simulink model "controller"  (Simulink 7.8)
settings: Solver=ode5  SolverMode=SingleTasking  StartTime=0.0  StopTime=50  FixedStep=0.01  RelTol=1e-3  AbsTol=1e-6
model workspace (MAT data in the model file):
  converter_data = [0  137.465208994  2.232; 0.1  137.065019157  2.075; 0.2  135.864449646  1.975; 0.3  135.664354728  1.846; 0.4  137.565256453  1.72; 0.5  140.366585312  1.564; 0.6  145.268910814  1.409; 0.7  152.872517717  1.254; 0.8  162.9773111  1.096; 0.81  164.27792807  1.08; 0.82  166.178829795  1.061; 0.83  167.979684062  1.043; 0.84  170.080680706  1.028; 0.85  172.781962105  1.012; 0.86  175.383196045  1.002; 0.87  179.585189333  1.002; 0.88  183.587087703  1.001; 0.89  189.890077635  0.998; 0.9  197.693779455  0.999; 0.92  215.902417037  1.001; 0.94  244.515990379  1.002]
  emap = [-40  -44  -49  -53  -57  -61  -65  -70  -74  -78  -82; 215  117  85  66  44  29  10  -2  -13  -22  -32; 245  208  178  148  122  104  85  66  48  33  18; 264  260  241  219  193  167  152  133  119  96  85; 264  279  282  275  260  238  223  208  189  171  152; 267  290  293  297  290  275  260  256  234  212  193; 267  297  305  305  305  301  293  282  267  249  226; 267  301  308  312  319  323  319  316  297  279  253; 267  301  312  319  327  327  327  327  312  293  267; 267  301  312  319  327  334  334  334  319  305  275]
  Iei = 0.0219914882836
  nevec = [800 1200 1600 2000 2400 2800 3200 3600 4000 4400 4800]
  p0 = 0.07934
  p1 = 0.07934
  thvec = [0; 20; 30; 40; 50; 60; 70; 80; 90; 100]
  vehicledata : num (value not decoded)
values from neighbouring files (symbols this model uses):
  downtab = [0 5 20 35 ... (first row only)    [transmission_data.m]
  downth = [0; 5; 40; 50; 90; 100]    [transmission_data.m]
  uptab = [10 30 50 1.0E+6 ... (first row only)    [transmission_data.m]
  upth = [0; 25; 35; 50; 90; 100]    [transmission_data.m]
Description:
  | ƒRƒ“ƒgƒ??[ƒ‰?eƒ‚ƒfƒ‹
settings Model: Creator=The MathWorks Inc.  LastModifiedBy=itoy  CovMetricSettings=dcmtr  CovHTMLOptions=-aTS=1 -bRG=1 -bTC=1 -hTR=0 -nFC=0 -scm=1 -bcm=1 -xEv=0  ExtModeTrigMode=oneshot  ExtModeArmWhenConnect=off  ExtModeAutoUpdateStatusClock=off
settings DataIOCC: LimitDataPoints=off  SaveOutput=off  SaveTime=off  SignalLoggingName=sigsOut
settings OptimizationCC: InlineParams=on  UseIntDivNetSlope=on  InlineInvariantSignals=on  InitFltsAndDblsToZero=on  EfficientMapNaN2IntZero=off  OptimizeModelRefInitCode=on  LifeSpan=1
settings DebuggingCC: SignalInfNanChecking=error  SaveWithParameterizedLinksMsg=none  CheckExecutionContextPreStartOutputMsg=on  CheckExecutionContextRuntimeOutputMsg=on  SolverPrmCheckMsg=none  MultiTaskDSMMsg=warning  MultiTaskCondExecSysMsg=none  IntegerOverflowMsg=error  FcnCallInpInsideContextMsg=Use local settings  BusObjectLabelMismatch=error  RootOutportRequireBusObject=error  StrictBusMsg=ErrorOnBusTreatedAsVector  BusNameAdapt=ErrorWithoutRepair  NonBusSignalsTreatedAsBus=error
settings HardwareCC: ProdIntDivRoundTo=Zero  ProdEndianess=LittleEndian  ProdHWDeviceType=NEC->V850  TargetIntDivRoundTo=Zero  TargetEndianess=LittleEndian  TargetHWDeviceType=MATLAB Host
settings ModelReferenceCC: ModelReferenceNumInstancesAllowed=Single
settings SFSimCC: SFSimEcho=off  SimParseCustomCode=off
settings RTWCC: SystemTargetFile=ert.tlc  TemplateMakefile=ert_default_tmf  Description=Embedded Coder  ProcessScript=ert_make_rtw_hook  IncludeERTFirstTime=on
settings CodeAppCC: IgnoreCustomStorageClasses=off  IgnoreTestpoints=on
settings ERTTargetCC: MultiwordLength=2048  GenerateSampleERTMain=on  IncludeMdlTerminateFcn=off  CombineSignalStateStructs=on  SuppressErrorStatus=on  SupportNonFinite=off  SupportComplex=off  PortableWordSizes=on  GenerateErtSFunction=on  CreateSILPILBlock=SIL  InlinedParameterPlacement=NonHierarchical  ERTCustomFileTemplate=example_file_process.tlc  ConvertIfToSwitch=off  SuppressUnreachableDefaultCases=off
settings ConfigComp: Description=Design Verifier Custom Configuration Component  DVMaxProcessTime=3000  DVModelCoverageObjectives=MCDC  DVMaxTestCaseSteps=500  DVTestSuiteOptimization=CombinedObjectives

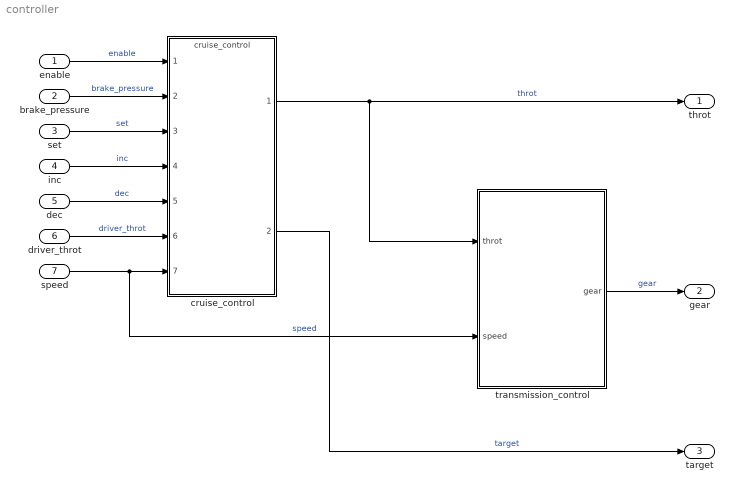
== system controller ==
  enable : Inport  PortDimensions=1
  brake_pressure : Inport  Port=2  PortDimensions=1
  set : Inport  Port=3  PortDimensions=1
  inc : Inport  Port=4  PortDimensions=1
  dec : Inport  Port=5  PortDimensions=1
  driver_throt : Inport  Port=6  PortDimensions=1
  speed : Inport  Port=7  PortDimensions=1
  cruise_control : ModelReference  ModelNameDialog=cruise_control  SimulationMode=Normal  ModelReferenceVersion=1.246  CopyOfModelName=cruise_control  DefaultDataLogging=off
  transmission_control : Subsystem  TreatAsAtomicUnit=on
  throt : Outport  PortDimensions=1
  gear : Outport  Port=2  PortDimensions=1
  target : Outport  Port=3  PortDimensions=1
  wires:
  speed/1 -> transmission_control/2(speed), cruise_control/7  "speed"
  driver_throt/1 -> cruise_control/6  "driver_throt"
  dec/1 -> cruise_control/5  "dec"
  inc/1 -> cruise_control/4  "inc"
  set/1 -> cruise_control/3  "set"
  brake_pressure/1 -> cruise_control/2  "brake_pressure"
  enable/1 -> cruise_control/1  "enable"
  transmission_control/1(gear) -> gear/1  "gear"
  cruise_control/2 -> target/1  "target"
  cruise_control/1 -> transmission_control/1(throt), throt/1  "throt"

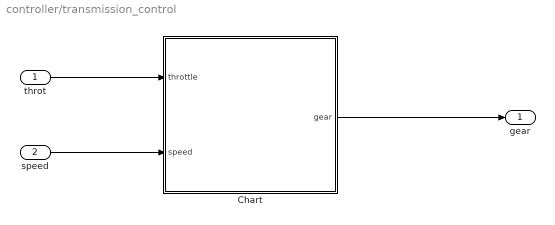
== system controller/transmission_control ==
  throt : Inport
  speed : Inport  Port=2
  Chart : Stateflow chart  TreatAsAtomicUnit=on
  gear : Outport
  wires:
  Chart/1(gear) -> gear/1
  speed/1 -> Chart/2(speed)
  throt/1 -> Chart/1(throttle)

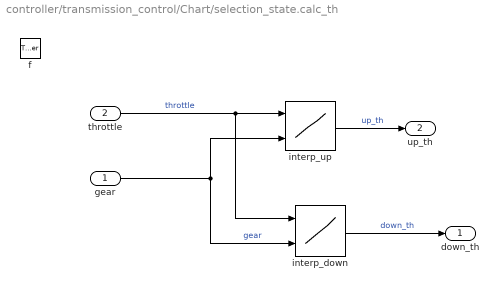
== system controller/transmission_control/Chart/selection_state.calc_th ==
  gear : Inport
  throttle : Inport  Port=2
  f : TriggerPort  TriggerType=function-call
      settings: CopyFcn=set_param(gcbh,'PreDeleteFcn','')  PreDeleteFcn=Stateflow.SLINSF.SimulinkMan.unsafePredeleteFcn
  interp_down : Lookup_n-D  BreakpointsForDimension1=downth  BreakpointsForDimension2=[1:4]  IndexSearchMethod=Linear search  Table=downtab  InterpMethod=Flat  ExtrapMethod=Clip  UseLastTableValue=on  InputSameDT=on
  interp_up : Lookup_n-D  BreakpointsForDimension1=upth  BreakpointsForDimension2=[1:4]  IndexSearchMethod=Linear search  Table=uptab  InterpMethod=Flat  ExtrapMethod=Clip  UseLastTableValue=on  InputSameDT=on
  down_th : Outport
  up_th : Outport  Port=2
  wires:
  gear/1 -> interp_down/2, interp_up/2  "gear"
  throttle/1 -> interp_down/1, interp_up/1  "throttle"
  interp_down/1 -> down_th/1  "down_th"
  interp_up/1 -> up_th/1  "up_th"

== stateflow chart transmission_control/Chart ==
  state gear_state [parallel]
    settings: executionOrder=1
    state fourth
      entry: gear = 4;
    state second
      entry: gear = 2;
    state third
      entry: gear = 3;
    state first
      entry: gear = 1;
    third -> fourth [order 2] : UP
    second -> third [order 2] : UP
    first -> second : UP
    (default) -> first
    fourth -> third : DOWN
    third -> second [order 1] : DOWN
    second -> first [order 1] : DOWN
  state selection_state [parallel]
    during: [down_th,up_th] = calc_th(gear,throttle);
    settings: executionOrder=2
    state downshifting
    state upshifting
    state steady_state
    state [down_th,up_th] = calc_th(gear,throttle) [function]
    (default) -> steady_state
    steady_state -> upshifting [order 1] : [speed > up_th]
    steady_state -> downshifting [order 2] : [speed < down_th && gear > 1]
    upshifting -> steady_state [order 2] : [speed < up_th]
    downshifting -> steady_state [order 2] : [speed > down_th]
    downshifting -> steady_state [order 1] : [after(TWAIT,tick) && speed <= down_th]
        | {gear_state.DOWN}
    upshifting -> steady_state [order 1] : [ after(TWAIT,tick) && speed >= up_th]
        | {gear_state.UP}
  data: gear function_input double; throttle function_input double; down_th function_output double; up_th function_output double; gear output uint16 [1..4] =1; TWAIT parameter uint8; up_th local double; down_th local double; throttle input double; speed input double
  events: DOWN local EITHER_EDGE_EVENT; UP local EITHER_EDGE_EVENT
